simulink model "qcg"  (R2024b)
settings: Solver=ode1  StartTime=0.0  StopTime=10  FixedStep=0.001  RelTol=1e-3
undefined symbols (not defined in the file): initial_qc_state, params
libraries: uavutilslib x3
settings Model: NumberOfSteps=10  Creator=William Riis  LastModifiedBy=William Riis

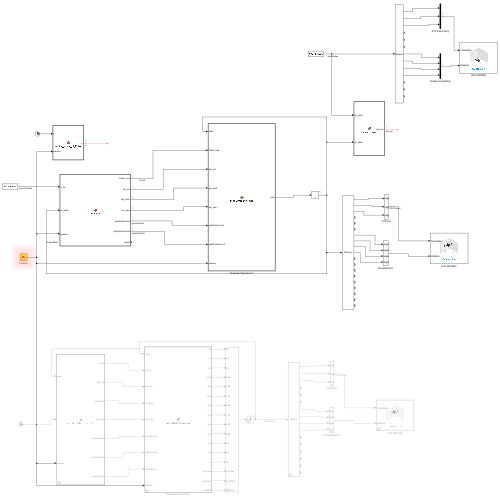
[thumbnail: Simulink's stored preview of the top-level diagram]
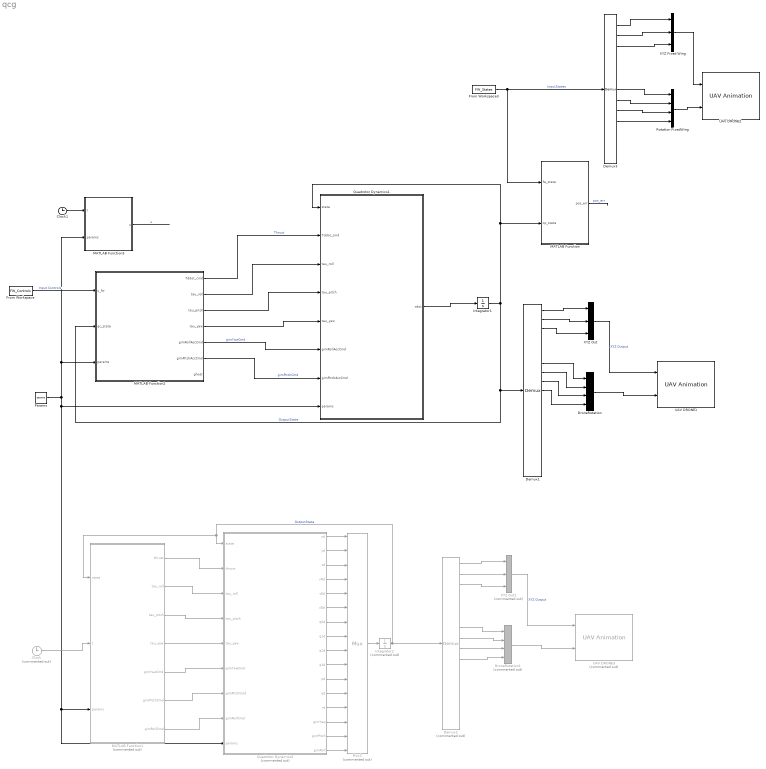
== system qcg ==
  Clock : Clock  Commented=on
  Clock1 : Clock
  Demux1 : Demux  Outputs=19
      settings: DisplayOption=none
  Demux2 : Demux  Commented=on  Outputs=16
      settings: DisplayOption=none
  Demux3 : Demux  Outputs=13
      settings: DisplayOption=none
  DroneRotation : Mux
      settings: DisplayOption=signals
  DroneRotation1 : Mux  Commented=on
      settings: DisplayOption=signals
  From Workspace : FromWorkspace  VariableName=FW_Controls  SampleTime=params.dt
  From Workspace3 : FromWorkspace  VariableName=FW_States  SampleTime=params.dt
  Integrator1 : Integrator  InitialCondition=initial_qc_state
  Integrator2 : Integrator  Commented=on  InitialCondition=initial_qc_state
  MATLAB Function : MATLAB Function  TreatAsAtomicUnit=on
  MATLAB Function1 : MATLAB Function  Commented=on  TreatAsAtomicUnit=on
  MATLAB Function2 : MATLAB Function  TreatAsAtomicUnit=on  SystemSampleTime=params.dt
  MATLAB Function3 : MATLAB Function  TreatAsAtomicUnit=on
  Mux2 : Mux  Commented=on  Inputs=16
      settings: DisplayOption=signals
  Params : Constant  Value=params  OutDataTypeStr=Bus: paramsBus
  Quadrotor Dynamics1 : MATLAB Function  TreatAsAtomicUnit=on
  Quadrotor Dynamics2 : MATLAB Function  Commented=on  TreatAsAtomicUnit=on
  Rotation FixedWing : Mux
  UAV DRONE1 : uavutilslib/UAV Animation  NumUAV=1  DynamicUAVConfig=off  UAVType=Multirotor  UAVSize=2  UAVColor=[1 0 1]  UAVTrajectoryAlpha=1  InertialZDirection=Down  RotationFormat=Quaternion  DrawMarkers=off  SampleTime=.01
  UAV DRONE2 : uavutilslib/UAV Animation  NumUAV=1  DynamicUAVConfig=off  UAVType=FixedWing  UAVSize=2  UAVColor=[0 0 0]  UAVTrajectoryAlpha=1  InertialZDirection=Down  RotationFormat=Quaternion  DrawMarkers=off  SampleTime=.01
  UAV DRONE3 : uavutilslib/UAV Animation  Commented=on  NumUAV=1  DynamicUAVConfig=off  UAVType=Multirotor  UAVSize=5  UAVColor=[0 0 1]  UAVTrajectoryAlpha=1  InertialZDirection=Down  RotationFormat=Quaternion  DrawMarkers=off  SampleTime=.01
  XYZ Fixed Wing : Mux  Inputs=3
  XYZ Out : Mux  Inputs=3
      settings: DisplayOption=signals
  XYZ Out1 : Mux  Commented=on  Inputs=3
      settings: DisplayOption=signals
  wires:
  Params/1 -> MATLAB Function1/3(params), Quadrotor Dynamics2/9(params), Quadrotor Dynamics1/8(params), MATLAB Function2/3(params), MATLAB Function3/2(params)
  Integrator1/1 -> Quadrotor Dynamics1/1(state), MATLAB Function/2(qc_state), MATLAB Function2/2(qc_state), Demux1/1  "OutputState"
  From Workspace3/1 -> Demux3/1, MATLAB Function/1(fw_state)  "InputStates"
  Demux3/3 -> XYZ Fixed Wing/3
  Demux3/2 -> XYZ Fixed Wing/2
  Demux3/1 -> XYZ Fixed Wing/1
  XYZ Out/1 -> UAV DRONE1/1  "XYZ Output"
  Demux1/1 -> XYZ Out/1
  Demux1/2 -> XYZ Out/2
  XYZ Fixed Wing/1 -> UAV DRONE2/1
  Rotation FixedWing/1 -> UAV DRONE2/2
  DroneRotation/1 -> UAV DRONE1/2
  Quadrotor Dynamics1/1(xdot) -> Integrator1/1
  Demux1/7 -> DroneRotation/1
  Demux1/8 -> DroneRotation/2
  Demux1/9 -> DroneRotation/3
  Demux1/10 -> DroneRotation/4
  MATLAB Function/1(pos_err) -> ?  "pos_err"
  Demux3/7 -> Rotation FixedWing/1
  Demux3/8 -> Rotation FixedWing/2
  Demux3/9 -> Rotation FixedWing/3
  Demux3/10 -> Rotation FixedWing/4
  Demux1/3 -> XYZ Out/3
  Quadrotor Dynamics2/16(gimRoll) -> Mux2/16
  Quadrotor Dynamics2/15(gimPitch) -> Mux2/15
  Quadrotor Dynamics2/14(gimYaw) -> Mux2/14
  Quadrotor Dynamics2/13(rd) -> Mux2/13
  Quadrotor Dynamics2/12(qd) -> Mux2/12
  Quadrotor Dynamics2/11(pd) -> Mux2/11
  Quadrotor Dynamics2/10(q3d) -> Mux2/10
  Quadrotor Dynamics2/9(q2d) -> Mux2/9
  Quadrotor Dynamics2/8(q1d) -> Mux2/8
  Quadrotor Dynamics2/7(q0d) -> Mux2/7
  Quadrotor Dynamics2/6(vDd) -> Mux2/6
  Quadrotor Dynamics2/4(vNd) -> Mux2/4
  Quadrotor Dynamics2/5(vEd) -> Mux2/5
  Quadrotor Dynamics2/3(zd) -> Mux2/3
  Quadrotor Dynamics2/2(yd) -> Mux2/2
  Quadrotor Dynamics2/1(xd) -> Mux2/1
  Mux2/1 -> Integrator2/1
  Demux2/3 -> XYZ Out1/3
  Demux2/10 -> DroneRotation1/4
  Demux2/9 -> DroneRotation1/3
  Demux2/8 -> DroneRotation1/2
  Demux2/7 -> DroneRotation1/1
  DroneRotation1/1 -> UAV DRONE3/2
  Demux2/2 -> XYZ Out1/2
  Demux2/1 -> XYZ Out1/1
  XYZ Out1/1 -> UAV DRONE3/1  "XYZ Output"
  Integrator2/1 -> Quadrotor Dynamics2/1(state), MATLAB Function1/1(state), Demux2/1  "OutputState"
  MATLAB Function1/1(thrust) -> Quadrotor Dynamics2/2(thrust)
  MATLAB Function1/2(tau_roll) -> Quadrotor Dynamics2/3(tau_roll)
  MATLAB Function1/3(tau_pitch) -> Quadrotor Dynamics2/4(tau_pitch)
  MATLAB Function1/4(tau_yaw) -> Quadrotor Dynamics2/5(tau_yaw)
  MATLAB Function1/5(gimYawCmd) -> Quadrotor Dynamics2/6(gimYawCmd)
  MATLAB Function1/6(gimPitchCmd) -> Quadrotor Dynamics2/7(gimPitchCmd)
  MATLAB Function1/7(gimRollCmd) -> Quadrotor Dynamics2/8(gimRollCmd)
  Clock/1 -> MATLAB Function1/2(t)
  MATLAB Function2/1(Tddot_cmd) -> Quadrotor Dynamics1/2(Tddot_cmd)  "Thrust"
  MATLAB Function2/2(tau_roll) -> Quadrotor Dynamics1/3(tau_roll)
  MATLAB Function2/3(tau_pitch) -> Quadrotor Dynamics1/4(tau_pitch)
  MATLAB Function2/4(tau_yaw) -> Quadrotor Dynamics1/5(tau_yaw)
  Clock1/1 -> MATLAB Function3/1(t)
  MATLAB Function3/1(u) -> ?  "u"
  MATLAB Function2/5(gimRollAccCmd) -> Quadrotor Dynamics1/6(gimRollAccCmd)  "gimYawCmd"
  MATLAB Function2/6(gimPitchAccCmd) -> Quadrotor Dynamics1/7(gimPitchAccCmd)  "gimPitchCmd"
  From Workspace/1 -> MATLAB Function2/1(u_fw)  "Input Controls"

== matlab function qcg/Quadrotor Dynamics2 ==
  data: state input; thrust input; tau_roll input; tau_pitch input; tau_yaw input; gimYawCmd input; gimPitchCmd input; gimRollCmd input; xd output; params input; yd output; zd output; vNd output; vEd output; vDd output; q0d output; q1d output; q2d output; q3d output; pd output; qd output; rd output; gimYaw output; gimPitch output; gimRoll output
function [xd,yd,zd, vNd,vEd,vDd, q0d,q1d,q2d,q3d, pd,qd,rd, gimYaw,gimPitch,gimRoll] = ...
    quadGimbalDynamics(state, thrust, tau_roll, tau_pitch, tau_yaw, ...
                       gimYawCmd, gimPitchCmd, gimRollCmd, params) %#codegen
% Quadrotor (NED, quaternion) + ideal 3-axis gimbal (algebraic pass-through)
% State(13): [x y z vN vE vD q0 q1 q2 q3 p q r]
% Inputs:
%   thrust [N] (along -b_z), tau_* [N·m] body torques,
%   gim*Cmd [rad] (desired gimbal yaw/pitch/roll from M-block),
%   params bus/struct
% Outputs:
%   13 derivatives + gimbal [yaw pitch roll] (rad), algebraic

% ---- Unpack state
vN = state(4); vE = state(5); vD = state(6);
q0 = state(7); q1 = state(8); q2 = state(9); q3 = state(10);
p  = state(11); q = state(12); r = state(13);

% ---- Params
m   = params.qc_m;
J   = params.qc_J;
g   = params.g;
rho = params.rho;

if isfield(params,'wind_ned'),  wind_ned = params.wind_ned(:); else, wind_ned = [0;0;0]; end
if isfield(params,'qc_CdA'),    CdA = params.qc_CdA(:).';      else, CdA = [0.02 0.03 0.05]; end
if isfield(params,'qc_T_min'),  T_min = params.qc_T_min; else, T_min = 0; end
if isfield(params,'qc_T_max'),  T_max = params.qc_T_max; else, T_max = inf; end
if isfield(params,'qc_tau_max'),tau_max = params.qc_tau_max(:); else, tau_max = [inf;inf;inf]; end
if isfield(params,'gim_ang_max'),gim_max = params.gim_ang_max(:); else, gim_max = [inf;inf;inf]; end

% ---- Normalize quaternion
qn = sqrt(q0*q0 + q1*q1 + q2*q2 + q3*q3);
if qn < 1e-12, q0=1; q1=0; q2=0; q3=0; else, q0=q0/qn; q1=q1/qn; q2=q2/qn; q3=q3/qn; end

% ---- Rotations
R_ib = quat2dcm([q0 q1 q2 q3]);     % body -> NED
R_bi = R_ib.';                      % NED  -> body

% ---- Velocities & airspeed
v_ned     = [vN; vE; vD];
v_air_ned = v_ned - wind_ned;
v_air_b   = R_bi * v_air_ned;

% ---- Forces in BODY
T_cmd      = min(max(thrust, T_min), T_max);
F_thrust_b = [0; 0; -T_cmd];   % along -b_z

Fd_b = -0.5 * rho * [CdA(1)*v_air_b(1)*abs(v_air_b(1));
                     CdA(2)*v_air_b(2)*abs(v_air_b(2));
                     CdA(3)*v_air_b(3)*abs(v_air_b(3))];

% ---- Sum forces in NED (gravity is +g in NED z)
F_ned      = R_ib * (F_thrust_b + Fd_b) + m * [0; 0; g];

% ---- Translational dynamics (NED)
v_dot_ned   = F_ned / m;
pos_dot_ned = v_ned;

% ---- Rotational dynamics (BODY)
tau_cmd = [tau_roll; tau_pitch; tau_yaw];
tau_cmd = max(min(tau_cmd, tau_max), -tau_max);

omega   = [p; q; r];
omega_d = J \ ( tau_cmd - cross(omega, J*omega) );

% ---- Quaternion kinematics via Aerospace Toolbox
qdot = 0.5 * quatmultiply([q0 q1 q2 q3], [0 p q r]); % row quats

% ---- Ideal gimbal: clamp and pass-through commanded angles
gimYaw   = max(min(gimYawCmd,   gim_max(1)), -gim_max(1));
gimPitch = max(min(gimPitchCmd, gim_max(2)), -gim_max(2));
gimRoll  = max(min(gimRollCmd,  gim_max(3)), -gim_max(3));

% ---- Pack derivatives
xd  = pos_dot_ned(1);  yd  = pos_dot_ned(2);  zd  = pos_dot_ned(3);
vNd = v_dot_ned(1);    vEd = v_dot_ned(2);    vDd = v_dot_ned(3);
q0d = qdot(1);         q1d = qdot(2);         q2d = qdot(3);         q3d = qdot(4);
pd  = omega_d(1);      qd  = omega_d(2);      rd  = omega_d(3);
end

== matlab function qcg/MATLAB Function1 ==
  settings: updateMethod=DISCRETE
  data: state input; t input; thrust output; tau_roll output; tau_pitch output; tau_yaw output; gimYawCmd output; gimPitchCmd output; gimRollCmd output; params input
function [thrust, tau_roll, tau_pitch, tau_yaw, gimYawCmd, gimPitchCmd, gimRollCmd] = ...
    qc_hold_initial_pose_snp(state, t, params) %#codegen
% Snappy & precise hold-initial-pose controller (DISCRETE)
% Frames: NED (Z down). Quat scalar-first [q0 q1 q2 q3], body->NED.
% No use of "clamp" helpers; explicit min/max saturations only.

% ── Unpack state
x  = state(1); y  = state(2); z  = state(3);
vN = state(4); vE = state(5); vD = state(6);
q0 = state(7); q1 = state(8); q2 = state(9); q3 = state(10);
p  = state(11); q  = state(12); r  = state(13);
gimYaw = state(14); gimPitch = state(15); gimRoll = state(16);

pos  = [x;y;z];
vel  = [vN;vE;vD];
quat = [q0 q1 q2 q3];
pqr  = [p;q;r];

% ── Params
m        = params.qc_m;
g        = params.g;
T_min    = getfield_or(params,'qc_T_min',0);
T_max    = getfield_or(params,'qc_T_max',inf);
tau_max  = getfield_or(params,'qc_tau_max',[inf;inf;inf]);

% Gains (snappy defaults; override in params)
Kp_xy    = getfield_or(params,'qc_Kp_xy',   3.0);
Ki_xy    = getfield_or(params,'qc_Ki_xy',   0.6);
Kd_xy    = getfield_or(params,'qc_Kd_xy',   1.2);

Kp_z     = getfield_or(params,'qc_Kp_z',    4.0);
Ki_z     = getfield_or(params,'qc_Ki_z',    2.0);
Kd_z     = getfield_or(params,'qc_Kd_z',    1.2);

Kp_ang   = getfield_or(params,'qc_Kp_ang',  [8.0; 8.0; 5.0]);
Kd_ang   = getfield_or(params,'qc_Kd_ang',  [2.0; 2.0; 1.2]);

% Limits
amax_xy  = getfield_or(params,'qc_amax_xy', 6.0);                % m/s^2 per-axis
amax_z   = getfield_or(params,'qc_amax_z',  4.0);                % m/s^2 (pre-g)
tilt_max = getfield_or(params,'qc_tilt_max_rad', deg2rad(25));   % rad
slew_a   = getfield_or(params,'qc_accel_slew', 30.0);            % m/s^3

% Sample time
dt_param = getfield_or(params,'dt', -1);
persistent last_t
dt = dt_param;
if ~(isnumeric(dt) && isscalar(dt) && dt > 0)
    if isempty(last_t), last_t = t; end
    dt = t - last_t; if ~isfinite(dt) || dt <= 0, dt = 0; end
end
last_t = t;

% ── Latch initial pose/yaw; integrators & slew states (DISCRETE)
persistent pos_ref xhat_yaw0 int_xy int_z a_cmd_prev initialized
if isempty(initialized)
    pos_ref     = pos;                       % hold initial [x0;y0;z0]
    R0          = quat2dcm(quat);            % body->NED at t0
    yaw0        = atan2(R0(2,1), R0(1,1));   % initial heading
    xhat_yaw0   = [cos(yaw0); sin(yaw0); 0];
    int_xy      = [0;0];
    int_z       = 0;
    a_cmd_prev  = [0;0;0];
    initialized = true;
end

% Anti-windup caps (in m*s)
I_xy_lim = getfield_or(params,'qc_I_xy_lim', 1.0);
I_z_lim  = getfield_or(params,'qc_I_z_lim',  2.0);

% ── Errors (NED)
e_pos = pos_ref - pos;   % z>0 ⇒ need to go DOWN
e_vel = -vel;

% ── Outer-loop PD+I → desired accel (NED)
a_xy = [ Kp_xy*e_pos(1) + Ki_xy*int_xy(1) + Kd_xy*e_vel(1);
         Kp_xy*e_pos(2) + Ki_xy*int_xy(2) + Kd_xy*e_vel(2) ];
a_z  =   Kp_z *e_pos(3) + Ki_z *int_z      + Kd_z *e_vel(3);

% Per-axis accel limits (avoid indexing errors)
a_xy(1) = min(max(a_xy(1), -amax_xy), amax_xy);
a_xy(2) = min(max(a_xy(2), -amax_xy), amax_xy);
a_z     = min(max(a_z,     -amax_z ), amax_z );

% Gravity compensation
a_cmd_des = [a_xy; a_z + g];

% Slew-limit accel command (per-axis)
if dt > 0
    a_delta_max = slew_a * dt;
    a_cmd = a_cmd_prev;
    for i = 1:3
        d = a_cmd_des(i) - a_cmd_prev(i);
        if d >  a_delta_max, d =  a_delta_max; end
        if d < -a_delta_max, d = -a_delta_max; end
        a_cmd(i) = a_cmd_prev(i) + d;
    end
else
    a_cmd = a_cmd_des;
end
a_cmd_prev = a_cmd;

% Update integrators AFTER limiting (discrete)
if dt > 0
    int_xy = int_xy + e_pos(1:2)*dt;
    % saturate integrator (per element)
    int_xy(1) = min(max(int_xy(1), -I_xy_lim), I_xy_lim);
    int_xy(2) = min(max(int_xy(2), -I_xy_lim), I_xy_lim);

    int_z  = int_z  + e_pos(3)*dt;
    int_z  = min(max(int_z,      -I_z_lim ),  I_z_lim );
end

% ── Desired force (NED)
F_des_ned = m * a_cmd;

% ── Current attitude
R_ib = quat2dcm(quat);      % body -> NED
R_bi = R_ib';

% ── Thrust along -b_z
F_b    = R_bi * F_des_ned;
T_req  = -F_b(3);
thrust = min(max(T_req, T_min), T_max);

% Simple back-calc anti-windup on vertical integrator if thrust limited
if T_req ~= thrust
    aw = 0.2;
    int_z = (1 - aw)*int_z;
end

% ── Desired attitude from desired force, keep initial yaw
% Desired -b_z direction:
if norm(F_des_ned) < 1e-6
    z_b_des = R_ib(:,3);
else
    z_b_des = -F_des_ned / max(norm(F_des_ned),1e-9);
end

% Enforce tilt limit: z component >= cos(tilt_max)
c = cos(tilt_max);
if z_b_des(3) < c
    h = z_b_des(1:2);
    nh = sqrt(h(1)^2 + h(2)^2);
    if nh > 1e-6
        h = h / nh;
        z_b_des = [h*sqrt(1 - c^2); c];
    else
        z_b_des = [0;0;1];
    end
end

% Build desired frame with initial heading
x_proj  = xhat_yaw0;                 % fixed heading vector (horizontal)
y_b_des = cross(z_b_des, x_proj);
ny = sqrt(sum(y_b_des.^2));
if ny < 1e-6
    x_proj  = [1;0;0];
    y_b_des = cross(z_b_des, x_proj);
    ny = sqrt(sum(y_b_des.^2));
end
y_b_des = y_b_des / ny;
x_b_des = cross(y_b_des, z_b_des);
R_des   = [x_b_des y_b_des z_b_des];

% ── SO(3) attitude error + rate damping → torques
E   = R_des' * R_ib - R_ib' * R_des;
e_R = 0.5 * [E(3,2) - E(2,3);
             E(1,3) - E(3,1);
             E(2,1) - E(1,2)];

tau_cmd = [ Kp_ang(1)*e_R(1) - Kd_ang(1)*pqr(1);
            Kp_ang(2)*e_R(2) - Kd_ang(2)*pqr(2);
            Kp_ang(3)*e_R(3) - Kd_ang(3)*pqr(3) ];

% Torque limits
tau_roll  = min(max(tau_cmd(1), -tau_max(1)), tau_max(1));
tau_pitch = min(max(tau_cmd(2), -tau_max(2)), tau_max(2));
tau_yaw   = min(max(tau_cmd(3), -tau_max(3)), tau_max(3));

% ── Gimbal passthrough (unchanged)
gimYawCmd   = gimYaw;
gimPitchCmd = gimPitch;
gimRollCmd  = gimRoll;

end

% ───────────────────────── helpers ─────────────────────────
function val = getfield_or(s, name, defaultVal)
if isfield(s, name); val = s.(name); else; val = defaultVal; end
end

== matlab function qcg/MATLAB Function3 ==
  data: t input; u output; params input
function u = control_inputs_bigPulse(t, params)
% 4x1 [ΔT; ΔE; ΔA; ΔR], pulses at 1.0, 1.2, 1.4, 1.6 s
% larger amplitudes to push beyond small-angle region
dt = double(params.dt);
u  = zeros(4,1);
ang = deg2rad(15);     % 15 deg surfaces
dT  = 0.30;            % +0.30 throttle
w   = 10*dt;           % 10-sample pulse width (short & punchy)
t0  = 1.0;

if t>=t0           && t<t0+w,         u(2) = +ang; end % Elevator @1.0s
if t>=t0+0.2      && t<t0+0.2+w,     u(3) = +ang; end % Aileron  @1.2s
if t>=t0+0.4      && t<t0+0.4+w,     u(4) = +ang; end % Rudder   @1.4s
if t>=t0+0.6      && t<t0+0.6+w,     u(1) = +dT;  end % Throttle @1.6s
end

== matlab function qcg/MATLAB Function2 ==
  data: u_fw input; qc_state input; params input; Tddot_cmd output; tau_roll output; tau_pitch output; tau_yaw output; gimRollAccCmd output; gimPitchAccCmd output; ghost output
function [Tddot_cmd, tau_roll, tau_pitch, tau_yaw, gimRollAccCmd, gimPitchAccCmd, ghost] = ...
    M_block(u_fw, qc_state, params)
% M_BLOCK  Differential-Flatness / NDI mapper: FW inputs -> QC+g commands
%
% Inputs
%   u_fw      : [thrust, elevator, aileron, rudder] (FW control inputs)
%   qc_state  : 19x1 QC+g state:
%               [x y z vN vE vD q0 q1 q2 q3 p q r T nu_T eta theta_g eta_dot theta_g_dot]'
%   params    : struct (see fields below)
%
% Outputs
%   Tddot_cmd       : commanded T̈ (N/s^2)
%   tau_roll/pitch/yaw : body torques (N·m)
%   gimRollAccCmd   : η̈ command (rad/s^2)
%   gimPitchAccCmd  : θ̈_g command (rad/s^2)
%   ghost           : struct with ghost FW refs (position, vel, a*, j*, s*, psi*, etc.)
%
% Key params (defaults used if absent):
%   dt, g, m_qc, J_qc (diag), tau_max (3x1)
%   k0_pos..k3_pos (pos chain), kpsi0,kpsi1 (yaw chain)
%   dfl.lambda0, dfl.lambda_b3, dfl.lambda_T  (ridge LS)
%   ghost_alpha_acc, ghost_alpha_jerk         (smoothing)
%   kg0_roll, kg1_roll, kg0_pitch, kg1_pitch  (gimbal PD)
%   fw_init_state (13x1), resetFW (bool)
%
% Notes
%   • Ghost FW is advanced here internally (RK4) and never reads the real FW sim.
%   • QC translational model assumes no drag (matches paper’s validation setup).

% ---------- unpack QC state
xq = qc_state(1); yq = qc_state(2); zq = qc_state(3);
vN = qc_state(4); vE = qc_state(5); vD = qc_state(6);
qBN_qc = qc_state(7:10);
p = qc_state(11); q = qc_state(12); r = qc_state(13);
T = qc_state(14);
nu_T = qc_state(15);
eta = qc_state(16); theta_g = qc_state(17);
eta_dot = qc_state(18); theta_g_dot = qc_state(19);

% ---------- params & defaults
dt  = getdef(params,'dt',0.001);
g   = getdef(params,'g',9.81);
m   = getdef(params,'m_qc',1.0);
J   = getdef(params,'J_qc',diag([0.02 0.02 0.035]));
Jx = J(1,1); Jy = J(2,2); Jz = J(3,3);
tau_lim = getdef(params,'tau_max',[1.2;1.2;1.2]);

k0 = getdef(params,'k0_pos',8.0);
k1 = getdef(params,'k1_pos',8.0);
k2 = getdef(params,'k2_pos',5.0);
k3 = getdef(params,'k3_pos',3.0);

kpsi0 = getdef(params,'kpsi0',6.0);
kpsi1 = getdef(params,'kpsi1',3.0);

lam0   = getdef_nested(params,'dfl','lambda0',1e-6);
lam_b3 = getdef_nested(params,'dfl','lambda_b3',1e-2);
lam_T  = getdef_nested(params,'dfl','lambda_T',0);

alpha_a = getdef(params,'ghost_alpha_acc',0.35);   % 0..1 (higher = less smoothing)
alpha_j = getdef(params,'ghost_alpha_jerk',0.35);

kg0_r = getdef(params,'kg0_roll',80.0);
kg1_r = getdef(params,'kg1_roll',20.0);
kg0_p = getdef(params,'kg0_pitch',80.0);
kg1_p = getdef(params,'kg1_pitch',20.0);

% ---------- persistent ghost buffers
persistent gSt gVelN_prev gAccN_prev gJerkN_prev psi_prev psidot_prev initd
if isempty(initd) || getdef(params,'resetFW',false)
    gSt = getdef(params,'fw_init_state',zeros(13,1));  % [x y z u v w q0 q1 q2 q3 p q r]'
    gVelN_prev  = zeros(3,1);
    gAccN_prev  = zeros(3,1);
    gJerkN_prev = zeros(3,1);
    psi_prev    = 0;
    psidot_prev = 0;
    initd = true;
end

% ---------- advance ghost FW one dt (RK4) using the same u_fw
% u_fw = [thrust, elevator, aileron, rudder]
k1 = fw_6dof_quat(gSt,       u_fw(1), u_fw(2), u_fw(3), u_fw(4), params);
k2 = fw_6dof_quat(gSt+0.5*dt*k1, u_fw(1), u_fw(2), u_fw(3), u_fw(4), params);
k3 = fw_6dof_quat(gSt+0.5*dt*k2, u_fw(1), u_fw(2), u_fw(3), u_fw(4), params);
k4 = fw_6dof_quat(gSt+dt*k3,     u_fw(1), u_fw(2), u_fw(3), u_fw(4), params);
gSt = gSt + dt*(k1 + 2*k2 + 2*k3 + k4)/6;

% normalize ghost quaternion (indices 7:10)
gSt(7:10) = gSt(7:10) / norm(gSt(7:10));

% ---------- ghost references in NED
xg = gSt(1); yg = gSt(2); zg = gSt(3);
ug = gSt(4); vg = gSt(5); wg = gSt(6);
qBN_g = gSt(7:10);
pg = gSt(11); qg = gSt(12); rg = gSt(13);

R_BN_g = quatNED_to_body(qBN_g);   % N->B
R_NB_g = R_BN_g.';
vN_g   = R_NB_g * [ug; vg; wg];    % ghost velocity in NED

% finite-diff ghost a*, j*, s* with smoothing
aN_g_raw = (vN_g - gVelN_prev)/dt;
jN_g_raw = (aN_g_raw - gAccN_prev)/dt;
sN_g_raw = (jN_g_raw - gJerkN_prev)/dt;

aN_g = (1-alpha_a)*gAccN_prev + alpha_a*aN_g_raw;
jN_g = (1-alpha_j)*gJerkN_prev + alpha_j*jN_g_raw;
sN_g = sN_g_raw;  % optional extra smoothing if desired

gVelN_prev  = vN_g;
gAccN_prev  = aN_g;
gJerkN_prev = jN_g;

% ghost yaw, yaw rate, yaw accel
psi_g     = yaw_from_RNB(R_NB_g);
psidot_g  = [0 0 1]* (R_NB_g * [pg;qg;rg]);
psiddot_g = (psidot_g - psidot_prev)/dt;
psi_prev    = psi_g;
psidot_prev = psidot_g;

% ---------- QC current kinematics needed for decoupling
R_BN = quatNED_to_body(qBN_qc);  % N->B
R_NB = R_BN.';
b3   = R_NB(:,3);                % body z-axis in N
b3dot = R_NB * [q; -p; 0];       % \dot b3 = R_NB * (omega x e3) with omega=[p;q;r]
% QC accel & jerk (model-based, no drag)
aN_qc = - (T/m)*b3 + [0;0;g];
jN_qc = - (nu_T/m)*b3 - (T/m)*b3dot;

% ---------- outer-loop shaping (4th-order position chain)
e_r = [xg;yg;zg] - [xq;yq;zq];
e_v = vN_g - [vN;vE;vD];
e_a = aN_g - aN_qc;
e_j = jN_g - jN_qc;

sN_cmd = sN_g + k3*e_j + k2*e_a + k1*e_v + k0*e_r;

% ---------- Build and solve translational 3×3 for [Tddot; tau_x; tau_y]
omega = [p;q;r];
Jomega = J*omega;

% helper for b3 second derivative term split:
% ddot b3 = R_NB*( omega × [q;-p;0] + M*J^{-1}(tau - omega×Jomega) )
Mmat = [0 1 0; -1 0 0; 0 0 0];
coupling_term = omega_cross(omega) * (R_NB(:,3)*0); %#ok<NASGU> % (not used; keeps notation)
% parts independent of tau:
ddotb3_bias = R_NB * ( cross(omega, [q;-p;0]) + Mmat*( J \ (-cross(omega,Jomega)) ) );

rhs = -m*sN_cmd ...
      - 2*b3dot*nu_T ...
      - T * ddotb3_bias;

% B matrix columns: [ b3 , (-T/Jx)R_NB(:,2) , (T/Jy)R_NB(:,1) ]
B = [ b3, (-T/Jx)*R_NB(:,2), (T/Jy)*R_NB(:,1) ];

% ridge parameter (conditioned by b3_z and T magnitude)
b3z = b3(3);
lambda = lam0 + lam_b3*(1 - b3z^2) + lam_T*( 1 / (1 + abs(T)) );

u_trans = ridge_ls(B, rhs, lambda);      % [Tddot; tau_x; tau_y]
Tddot_cmd = u_trans(1);
tau_x     = u_trans(2);
tau_y     = u_trans(3);

% ---------- Yaw channel (2nd-order): psï_cmd then tau_z
% current yaw & yaw rate
psi_qc    = yaw_from_RNB(R_NB);
psidot_qc = [0 0 1] * (R_NB * [p;q;r]);

e_psi   = wrapToPi(psi_g - psi_qc);
e_psid  = (psidot_g - psidot_qc);
psidd_cmd = psiddot_g + kpsi1*e_psid + kpsi0*e_psi;

% psï = e3^T R_NB J^{-1}(tau - omega×Jomega)
aPsi = [0 0 1] * R_NB * (J \ eye(3));     % 1x3 row
biasPsi = [0 0 1] * R_NB * (J \ (-cross(omega,Jomega)));

% subtract already-chosen tau_x,tau_y contribution to psï
psi_dd_from_xy = aPsi(1)*tau_x + aPsi(2)*tau_y;
den = aPsi(3);
if abs(den) < 1e-6
    tau_z = 0;  % near-singular, fall back to zero (or clamp)
else
    tau_z = (psidd_cmd - biasPsi - psi_dd_from_xy) / den;
end

% ---------- Saturate torques
tau = [tau_x; tau_y; tau_z];
tau = min(max(tau, -abs(tau_lim)), abs(tau_lim));
tau_roll  = tau(1);
tau_pitch = tau(2);
tau_yaw   = tau(3);

% ---------- Gimbal: make camera POV match ghost FW body frame
% Desired R_CB such that R_CB * R_BN_qc ≈ R_BN_g  →  R_CB_des = R_BN_g * R_NB_qc
R_CB_des = R_BN_g * R_NB;

% extract η*, θ*_g for R_CB = R_x(η) R_y(θ)
theta_des = atan2( -R_CB_des(1,3), R_CB_des(1,1) );
eta_des   = atan2( -R_CB_des(3,2), R_CB_des(2,2) );

% PD to produce joint accelerations (desired rates set to 0 here)
gimRollAccCmd  = kg0_r * wrapToPi(eta_des - eta)       + kg1_r * (0 - eta_dot);
gimPitchAccCmd = kg0_p * wrapToPi(theta_des - theta_g) + kg1_p * (0 - theta_g_dot);

% ---------- ghost struct for logging/plotting
ghost = struct();
ghost.rN   = [xg; yg; zg];
ghost.vN   = vN_g;
ghost.aN   = aN_g;
ghost.jN   = jN_g;
ghost.sN   = sN_g;
ghost.psi  = psi_g;
ghost.psidot  = psidot_g;
ghost.psiddot = psiddot_g;
ghost.R_NB_fw  = R_NB_g;
ghost.R_CB_des = R_CB_des;

end
% ========================= helpers ==============================

function R = quatNED_to_body(q)
% q = [q0 q1 q2 q3] (scalar-first), mapping NED -> Body (Hamilton)
q0 = q(1); q1 = q(2); q2 = q(3); q3 = q(4);
R = [ 1-2*(q2^2+q3^2),   2*(q1*q2 + q0*q3),  2*(q1*q3 - q0*q2);
      2*(q1*q2 - q0*q3), 1-2*(q1^2+q3^2),    2*(q2*q3 + q0*q1);
      2*(q1*q3 + q0*q2), 2*(q2*q3 - q0*q1),  1-2*(q1^2+q2^2) ];
end

function y = yaw_from_RNB(R_NB)
% Extract ZYX yaw (about +Z_ned) from R_NB (body->NED)
% tan(psi) = R_NB(2,1) / R_NB(1,1)
y = atan2(R_NB(2,1), R_NB(1,1));
end

function u = ridge_ls(B, d, lambda)
% Solve (B'B + lambda I)u = B'd
BtB = B.'*B;
rhs = B.'*d;
u = (BtB + lambda*eye(size(BtB))) \ rhs;
end

function A = omega_cross(w)
% skew-symmetric matrix [w]x
A = [   0   -w(3)  w(2);
      w(3)    0   -w(1);
     -w(2)  w(1)    0  ];
end

function out = getdef(S, field, defaultVal)
if isfield(S, field), out = S.(field); else, out = defaultVal; end
end

function out = getdef_nested(S, f1, f2, defaultVal)
if isfield(S,f1) && isfield(S.(f1),f2), out = S.(f1).(f2); else, out = defaultVal; end
end

function ang = wrapToPi(ang)
% wrap angle(s) to [-pi,pi]
ang = mod(ang + pi, 2*pi) - pi;
end

== matlab function qcg/MATLAB Function ==
  data: fw_state input; pos_err output; qc_state input
function pos_err = compare_states(fw_state, qc_state)
% Position error only (NED): [x; y; z]_fw - [x; y; z]_qc
% fw_state: [x y z u v w q0 q1 q2 q3 p q r]
% qc_state: [x y z vN vE vD q0 q1 q2 q3 p q r gimYaw gimPitch gimRoll]
pos_err = fw_state(1:3) - qc_state(1:3);
end

== matlab function qcg/Quadrotor Dynamics1 ==
  data: state input; Tddot_cmd input; tau_roll input; tau_pitch input; tau_yaw input; gimRollAccCmd input; gimPitchAccCmd input; xdot output; params input
function xdot = quadGimbalDynamics(state, Tddot_cmd, tau_roll, tau_pitch, tau_yaw, ...
                                   gimRollAccCmd, gimPitchAccCmd, params)
% QUADGIMBALDYNAMICS  6-DoF quadrotor with thrust double-integrator + 2-axis gimbal
%
% State (19x1):
%   [x y z vN vE vD q0 q1 q2 q3 p q r T nu_T eta theta_g eta_dot theta_g_dot]'
% Inputs:
%   Tddot_cmd        : commanded T̈  (N/s^2)
%   tau_roll/pitch/yaw: body torques (N·m) about Bx,By,Bz
%   gimRollAccCmd    : commanded gimbal roll  acceleration η̈ (rad/s^2)
%   gimPitchAccCmd   : commanded gimbal pitch acceleration θ̈g (rad/s^2)
% Params (required fields; sensible defaults used if missing):
%   qc_m, qc_J, qc_T_min, qc_T_max, qc_tau_max (3x1), g, rho, dt
%   wind_ned (3x1), qc_CdA (1x3, NED axes)  [optional; default zeros]
%   gim_ang_max (2x1), gim_rate_max (2x1), gimbal_ideal (bool) [optional]
%
% Frames: NED (Z down). Total thrust acts along -z_B.
% Quaternion convention: scalar-first Hamilton, q_BN rotates NED→Body.

% -------- Unpack state
x     = state(1);  %#ok<NASGU>
y     = state(2);  %#ok<NASGU>
z     = state(3);  %#ok<NASGU>
vN    = state(4);
vE    = state(5);
vD    = state(6);
qBN   = state(7:10);     % [q0 q1 q2 q3], N->B
pqr   = state(11:13);    % [p q r] (rad/s), body rates
T     = state(14);       % total thrust (N)
nu_T  = state(15);       % Tdot (N/s)
eta   = state(16);       % gimbal roll about Bx (rad)
theta = state(17);       % gimbal pitch about By after Rx (rad)
etad  = state(18);       % η̇
thetad= state(19);       % θ̇g

% -------- Params & defaults
m   = getfield_def(params,'qc_m',1.0);
J   = getfield_def(params,'qc_J',diag([0.02 0.02 0.035]));
g   = getfield_def(params,'g',9.81);
rho = getfield_def(params,'rho',1.225);

Tmin = getfield_def(params,'qc_T_min',0);
Tmax = getfield_def(params,'qc_T_max',30);
tau_lim = getfield_def(params,'qc_tau_max',[1.2;1.2;1.2]);

CdA = getfield_def(params,'qc_CdA',[0 0 0]);     % per-axis (NED)
wind_ned = getfield_def(params,'wind_ned',[0;0;0]);

% (Optional) thrust rate/acc limits
Tdot_max  = getfield_def(params,'qc_Tdot_max',inf);
Tddot_max = getfield_def(params,'qc_Tddot_max',inf);

% Gimbal limits
gim_ang_max  = getfield_def(params,'gim_ang_max',deg2rad([60;45]));   % [roll; pitch]
gim_rate_max = getfield_def(params,'gim_rate_max',deg2rad([360;360]));
gim_acc_max  = getfield_def(params,'gim_acc_max',inf(2,1));           % optional
gimbal_ideal = getfield_def(params,'gimbal_ideal',false);

% -------- Rotation stuff
R_BN = quatNED_to_body(qBN);   % N -> B
R_NB = R_BN.';                 % B -> N
b3_N = R_NB(:,3);              % body z-axis expressed in NED

% -------- Kinematics (positions)
x_dot = vN;
y_dot = vE;
z_dot = vD;

% -------- Translational dynamics (NED)
vNED   = [vN; vE; vD];
v_air  = vNED - wind_ned;

% Thrust in NED: F_thrust = -T * b3_N
F_thrust_N = -T * b3_N;

% Quadratic drag per-axis in NED (optional; zero by default)
F_drag_N = -0.5 * rho * [CdA(1)*abs(v_air(1))*v_air(1);
                         CdA(2)*abs(v_air(2))*v_air(2);
                         CdA(3)*abs(v_air(3))*v_air(3)];

aNED = (F_thrust_N + F_drag_N)/m + [0;0;g];   % g is +down in NED

vN_dot = aNED(1);
vE_dot = aNED(2);
vD_dot = aNED(3);

% -------- Attitude kinematics (quaternion) & rotational dynamics
p = pqr(1); q = pqr(2); r = pqr(3);
q0 = qBN(1); q1 = qBN(2); q2 = qBN(3); q3 = qBN(4);

Omega = [ 0   -p   -q   -r;
          p    0    r   -q;
          q   -r    0    p;
          r    q   -p    0 ];
qBN_dot = 0.5 * Omega * [q0;q1;q2;q3];
% (Normalize q in the driver after integration.)

% Body torques with saturation
tau_cmd = [tau_roll; tau_pitch; tau_yaw];
tau     = saturate_vec(tau_cmd, tau_lim);

% Euler's equation
pqr_dot = J \ ( tau - cross(pqr, J*pqr) );

% -------- Thrust double integrator with conditional anti-windup
% Limit T̈ then apply basic boundary logic for Ṫ if T at limits.
Tdd = saturate_scalar(Tddot_cmd, -Tddot_max, Tddot_max);

% Prevent integrating past hard T limits
if (T >= Tmax && nu_T > 0 && Tdd >= 0), Tdd = 0; end
if (T <= Tmin && nu_T < 0 && Tdd <= 0), Tdd = 0; end

% Also limit Ṫ magnitude if provided
if isfinite(Tdot_max)
    if nu_T >=  Tdot_max && Tdd >  0, Tdd = 0; end
    if nu_T <= -Tdot_max && Tdd <  0, Tdd = 0; end
end

T_dot   = nu_T;
nu_Tdot = Tdd;

% -------- Gimbal joint dynamics (roll=η about Bx, pitch=θ about By after Rx)
eta_dd   = saturate_scalar(gimRollAccCmd,  -gim_acc_max(1),  gim_acc_max(1));
theta_dd = saturate_scalar(gimPitchAccCmd, -gim_acc_max(2),  gim_acc_max(2));

if ~gimbal_ideal
    % Rate limits (if at rate limit and trying to speed up further, block)
    if abs(etad)   >= gim_rate_max(1) && sign(eta_dd)   == sign(etad),   eta_dd   = 0; end
    if abs(thetad) >= gim_rate_max(2) && sign(theta_dd) == sign(thetad), theta_dd = 0; end

    % Angle soft stops: if beyond angle limit and still pushing outwards, damp it
    k_stop = 50;   % damping toward boundary when saturated
    if abs(eta) >= gim_ang_max(1) && sign(etad) == sign(eta)
        if sign(eta_dd) == sign(eta), eta_dd = -k_stop*etad; end
    end
    if abs(theta) >= gim_ang_max(2) && sign(thetad) == sign(theta)
        if sign(theta_dd) == sign(theta), theta_dd = -k_stop*thetad; end
    end
else
    % "Ideal" path: no extra limiting here (use very large limits in params)
end

% -------- Assemble xdot
xdot = zeros(19,1);
xdot(1)  = x_dot;
xdot(2)  = y_dot;
xdot(3)  = z_dot;
xdot(4)  = vN_dot;
xdot(5)  = vE_dot;
xdot(6)  = vD_dot;
xdot(7:10)  = qBN_dot;
xdot(11:13) = pqr_dot;
xdot(14) = T_dot;
xdot(15) = nu_Tdot;
xdot(16) = etad;
xdot(17) = thetad;
xdot(18) = eta_dd;
xdot(19) = theta_dd;

end

% ===================== helpers ==========================
function R = quatNED_to_body(q)
% q = [q0 q1 q2 q3] (scalar-first), mapping NED -> Body
q0 = q(1); q1 = q(2); q2 = q(3); q3 = q(4);
% Hamilton, passive, N->B
R = [ 1-2*(q2^2+q3^2),   2*(q1*q2 + q0*q3),  2*(q1*q3 - q0*q2);
      2*(q1*q2 - q0*q3), 1-2*(q1^2+q3^2),    2*(q2*q3 + q0*q1);
      2*(q1*q3 + q0*q2), 2*(q2*q3 - q0*q1),  1-2*(q1^2+q2^2) ];
end

function y = saturate_scalar(u, umin, umax)
y = min(max(u, umin), umax);
end

function y = saturate_vec(u, umax_vec)
% symmetric limits per axis: [-umax, +umax]
y = min(max(u, -abs(umax_vec)), abs(umax_vec));
end

function out = getfield_def(S, field, defaultVal)
if isfield(S, field), out = S.(field); else, out = defaultVal; end
end
